simulink model "gain2"  (R2022b)
settings: Solver=VariableStepAuto  StartTime=0.0  StopTime=100.0  RelTol=1e-3
settings Model: Creator=马飞  LastModifiedBy=acer
settings ModelReferenceCC: EnableRefExpFcnMdlSchedulingChecks=on

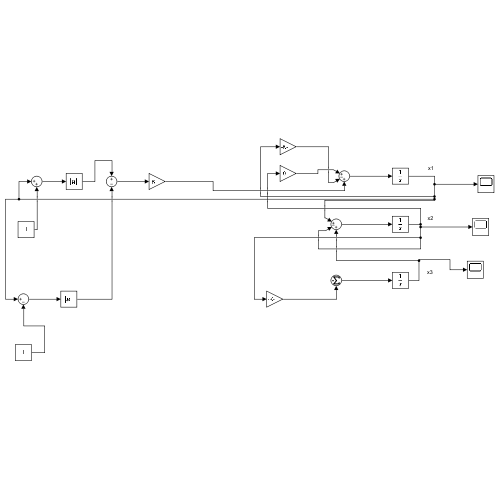
[thumbnail: Simulink's stored preview of the top-level diagram]
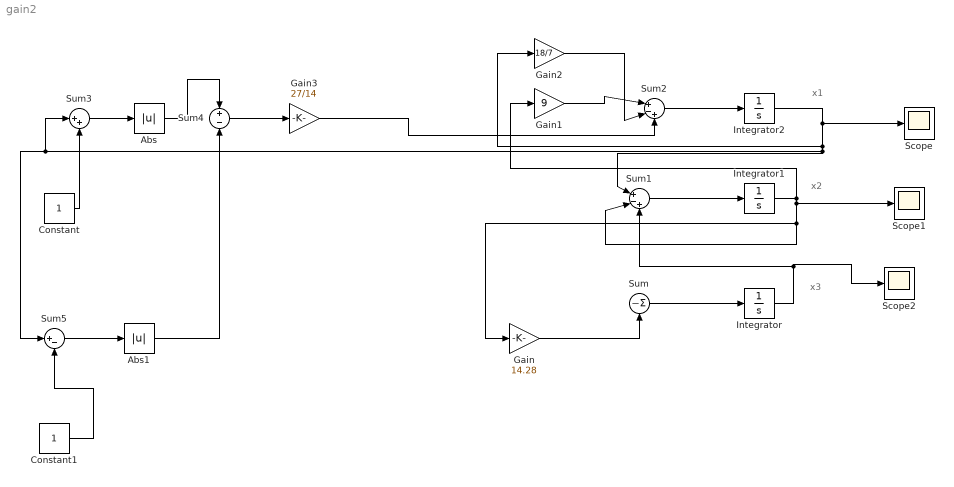
== system gain2 ==
  note: x3
  note: x2
  note: x1
  Abs : Abs  SaturateOnIntegerOverflow=off
  Abs1 : Abs  SaturateOnIntegerOverflow=off
  Constant : Constant
  Constant1 : Constant
  Gain : Gain  Gain=14.28
  Gain1 : Gain  Gain=9
  Gain2 : Gain  Gain=18/7
  Gain3 : Gain  Gain=27/14
  Integrator : Integrator  InitialCondition=0.7
  Integrator1 : Integrator  InitialCondition=0.3
  Integrator2 : Integrator  InitialCondition=-0.2
  Scope : Scope
  Scope1 : Scope
  Scope2 : Scope
  Sum : Sum  Inputs=|-
  Sum1 : Sum  Inputs=|+-+
  Sum2 : Sum  Inputs=|+-+
  Sum3 : Sum  Inputs=|++
  Sum4 : Sum  Inputs=+-
  Sum5 : Sum  Inputs=|+-
  wires:
  Integrator1/1 -> Sum1/2, Gain/1, Scope1/1, Gain1/1
  Integrator2/1 -> Scope/1, Sum5/1, Sum3/1, Sum1/1, Gain2/1
  Sum/1 -> Integrator/1
  Sum1/1 -> Integrator1/1
  Gain/1 -> Sum/1
  Sum2/1 -> Integrator2/1
  Gain1/1 -> Sum2/1
  Gain2/1 -> Sum2/2
  Constant/1 -> Sum3/2
  Sum3/1 -> Abs/1
  Abs/1 -> Sum4/1
  Constant1/1 -> Sum5/2
  Sum5/1 -> Abs1/1
  Abs1/1 -> Sum4/2
  Sum4/1 -> Gain3/1
  Gain3/1 -> Sum2/3
  Integrator/1 -> Scope2/1, Sum1/3
